simulink model "Reafference"  (R2015b)
settings: Solver=ode4  StartTime=0.0  StopTime=35.995  FixedStep=0.005  RelTol=1e-3
values from neighbouring files (symbols this model uses):
  delay = 0.25    [modelInit.m]    (also in modelInit_forward.m = 0.1)
  dt = 0.005    [modelInit.m]    (also in modelInit_forward.m)
  F = 2.0*(rand(N,dOut)-0.5)    [modelInit.m]    (also in modelInit_forward.m)
  I = 2.0*(rand(N,dIn)-0.5)    [modelInit.m]    (also in modelInit_forward.m)
  I_fore_x = infactor*(5.66+0.306*m_k-0.088*l_k)/10000    (= 0.0024252)    [modelInit.m]    (also in modelInit_forward.m)
  I_fore_y = infactor*(-64+0.95*m_k+0.34*l_k)/10000    (= 0.012004)    [modelInit.m]    (also in modelInit_forward.m)
  I_fore_z = infactor*(-67.9+0.855*m_k+0.376*l_k)/10000    (= 0.0112156)    [modelInit.m]    (also in modelInit_forward.m)
  I_hand_x = infactor*(-6.26+0.0762*m_k+0.0347*l_k)/10000    (= 0.00100322)    [modelInit.m]    (also in modelInit_forward.m)
  I_hand_y = infactor*(-19.5+0.17*m_k+0.116*l_k)/10000    (= 0.0024796)    [modelInit.m]    (also in modelInit_forward.m)
  I_hand_z = infactor*(-13.68+0.088*m_k+0.092*l_k)/10000    (= 0.0015832)    [modelInit.m]    (also in modelInit_forward.m)
  I_upper_x = (-16.9+0.662*m_k+0.0453*l_k)/10000    (= 0.00718718)    [modelInit.m]    (also in modelInit_forward.m)
  I_upper_y = (-250.7+1.56*m_k+1.512*l_k)/10000    (= 0.0247972)    [modelInit.m]    (also in modelInit_forward.m)
  I_upper_z = (-232+1.525*m_k+1.343*l_k)/10000    (= 0.0227658)    [modelInit.m]    (also in modelInit_forward.m)
  l_fore = 0.30    (= 0.3)    [modelInit.m]    (also in modelInit_forward.m)
  l_hand = 0.20    (= 0.2)    [modelInit.m]    (also in modelInit_forward.m)
  l_upper = 0.36    [modelInit.m]    (also in modelInit_forward.m)
  learn = 1    [modelLearn.m]    (also in modelLearn_forward.m; modelMorph.m = 0; modelMorph_forward.m = 0; modelVal.m = 0)
  M = full(sprandn(N,N,p)*g*1.0/sqrt(p*N))    [modelInit.m]    (also in modelInit_forward.m)
  m_fore = m_fore*wfactor    (= 1.81766)    [modelInit.m]    (also in modelInit_forward.m)
  m_hand = m_hand*wfactor    (= 0.676)    [modelInit.m]    (also in modelInit_forward.m)
  m_upper = m_upper*wfactor    (= 3.3082)    [modelInit.m]    (also in modelInit_forward.m)
  N = 1000    [modelInit.m]    (also in modelInit_forward.m)
  P0 = (1.0/alpha)*eye(N,N)    [modelInit.m]    (also in modelInit_forward.m; modelMorph.m = simOutLearn.get('P'); modelMorph_forward.m = simOutLearn.get('P'); modelVal.m = simOutLearn.get('P'))
  q0 = 0.5*randn(N,1)    [modelInit.m]    (also in modelInit_forward.m; modelMorph.m = simOutLearn.get('q'); modelMorph_forward.m = simOutLearn.get('q'); modelVal.m = simOutLearn.get('q'))
  tau = 0.01    [modelInit.m]    (also in modelInit_forward.m)
  W0 = zeros(dOut,N)    [modelInit.m]    (also in modelInit_forward.m; modelMorph.m = simOutLearn.get('W'); modelMorph_forward.m = simOutLearn.get('W'); modelVal.m = simOutLearn.get('W'))
undefined symbols (not defined in the file or in its folder): DiscIntNeverNeededParam, Muscle, MuscleLib, Newton, Raphson
undefined symbols (not defined in the file): bifactor, brfactor, trifactor
libraries: mblibv1 x26, simulink x3
settings Model: ExtModeTrigDuration=100  Creator=kbostroem  LastModifiedBy=kbostroem
settings DataIOCC: LimitDataPoints=off  SaveFinalState=on  SaveFormat=StructureWithTime  SignalLoggingSaveFormat=ModelDataLogs  SaveOutput=off  SaveState=on  StateSaveName=tmp_raccel_xout  SignalLoggingName=tmp_raccel_logsout  OutputTimes=linspace(0,20,1000)
settings OptimizationCC: ExpressionDepthLimit=2147483647  EfficientMapNaN2IntZero=off
settings DebuggingCC: UnderspecifiedInitializationDetection=Classic  MergeDetectMultiDrivingBlocksExec=none  SolverPrmCheckMsg=warning  FcnCallInpInsideContextMsg=EnableAllAsWarning  StateNameClashWarn=warning
settings HardwareCC: ProdBitPerPointer=32  ProdLargestAtomicFloat=None  ProdIntDivRoundTo=Undefined  ProdEndianess=Unspecified  ProdWordSize=32  ProdHWDeviceType=32-bit Generic  TargetBitPerLong=64  TargetBitPerPointer=64  TargetLongLongMode=on  TargetIntDivRoundTo=Zero  TargetEndianess=LittleEndian  TargetWordSize=64  TargetHWDeviceType=MATLAB Host  ProdEqTarget=off
settings RTWCC: SystemTargetFile=raccel.tlc  TemplateMakefile=raccel_default_tmf  RTWVerbose=off  RTWUseSimCustomCode=on
settings CodeAppCC: GenerateComments=off  MaxIdLength=128  MangleLength=10  SimulinkBlockComments=off
settings RaccelTargetCC: ERTMultiwordTypeDef=System defined  ERTMultiwordLength=256  GeneratePreprocessorConditionals=Disable all  ERTFirstTimeCompliant=off  MultiInstanceERTCode=off  ENABLE_SLEXEC_SSBRIDGE=0  RTWCAPIParams=off
settings ConfigComp: CovModelRefEnable=Off  CovSFcnEnable=off
settings SimscapeCC: SimscapeLogType=all  SimscapeLogDataHistory=10000
settings SimMechanicsCC: VisOnUpdateDiagram=on  LastVizWinPosition=[133 241 630 553]  CamPosition=[0.122075;1.72207;11.4539;]  CamTarget=[0.122075;1.72207;0;]  CamUpVector=[0;1;0;]  CamHeight=0.668977  VisBackgroundColor=[0.9;0.9;0.95;]  DefaultBodyColor=[1;0;0;]

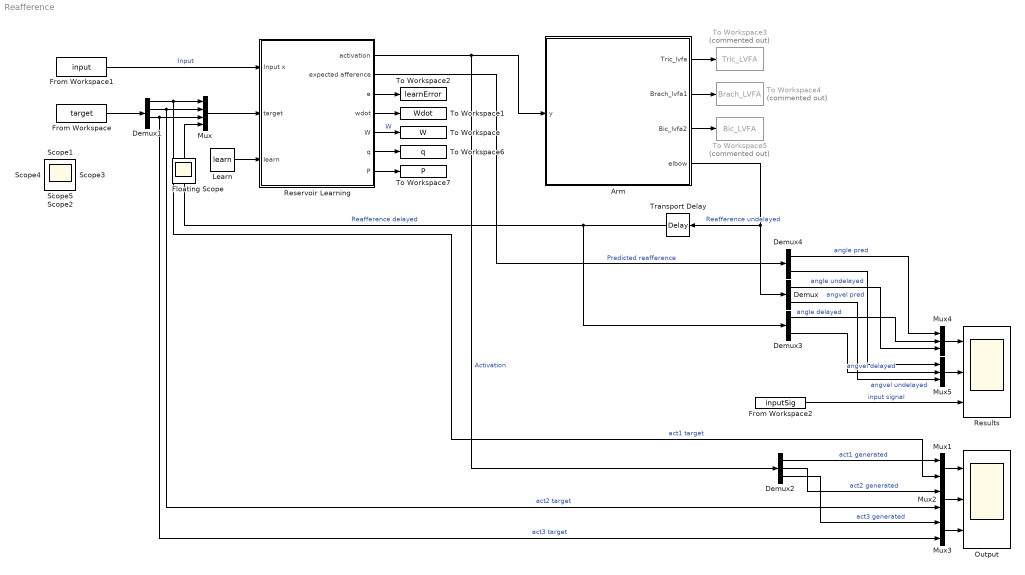
== system Reafference ==
  Arm : Subsystem
      mask Display:
      | image(imread('icons/ArmModell.jpg'));
      | 
      | port_label('output', 1, 'Tric_LVFA');
      | port_label('output', 2, 'Brach_LVFA');
      | port_label('output', 3, 'Bic_LVFA');
      | color('blue')
      | port_label('output', 4, 'Elbow Afference');
      | port_label('input', 1, 'Activation');
  Demux : Demux  Outputs=2
  Demux1 : Demux
  Demux2 : Demux  Outputs=3
  Demux3 : Demux  Outputs=2
  Demux4 : Demux  Outputs=2
  From Workspace : FromWorkspace  VariableName=target  SampleTime=dt  Interpolate=off  OutputAfterFinalValue=Cyclic repetition
  From Workspace1 : FromWorkspace  VariableName=input  SampleTime=dt  Interpolate=off  OutputAfterFinalValue=Cyclic repetition
  From Workspace2 : FromWorkspace  VariableName=inputSig  SampleTime=dt  Interpolate=off  OutputAfterFinalValue=Cyclic repetition
  Learn : Constant  Value=learn
  Mux : Mux
  Mux1 : Mux  Inputs=2
  Mux2 : Mux  Inputs=2
  Mux3 : Mux  Inputs=2
  Mux4 : Mux  Inputs=3
  Mux5 : Mux  Inputs=3
  Output : Scope  NumInputPorts=3
  Reservoir Learning : Subsystem
      mask Display:
      | image(imread('icons/liquidMotion.jpg'));
      | port_label('input', 1, 'Input x');
      | port_label('input', 2, 'Target h');
      | port_label('output', 1, 'Output y');
      | 
      | color('white')
      | port_label('input', 3, 'learn');
      | port_label('output', 2, 'Predicted reafference');
      | port_label('output', 3, 'error');
      | port_label('output', 4, 'w_dot');
      | port_label('output', 5, 'W');
      | port_label('output', 6, 'q');
      | port_label('output', 7, 'P');
  Results : Scope  NumInputPorts=3
  To Workspace : ToWorkspace  VariableName=W  SampleTime=-1
      settings: MaxDataPoints=1
  To Workspace1 : ToWorkspace  VariableName=Wdot  SampleTime=-1
      settings: MaxDataPoints=Inf
  To Workspace2 : ToWorkspace  VariableName=learnError  SampleTime=-1
      settings: MaxDataPoints=1
  To Workspace3 : ToWorkspace  Commented=on  VariableName=Tric_LVFA  SampleTime=-1
      settings: MaxDataPoints=Inf
  To Workspace4 : ToWorkspace  Commented=on  VariableName=Brach_LVFA  SampleTime=-1
      settings: MaxDataPoints=Inf
  To Workspace5 : ToWorkspace  Commented=on  VariableName=Bic_LVFA  SampleTime=-1
      settings: MaxDataPoints=Inf
  To Workspace6 : ToWorkspace  VariableName=q  SampleTime=-1
      settings: MaxDataPoints=1
  To Workspace7 : ToWorkspace  VariableName=P  SampleTime=-1
      settings: MaxDataPoints=1
  Transport Delay : TransportDelay  DelayTime=delay  InitialOutput=[130/180*pi; 0]
  Floating Scope : Scope
  Scope{,1..5} (6 alike) : Scope
  wires:
  Demux1/1 -> Mux1/2, Mux/1  "act1 target"
  Demux1/2 -> Mux2/2, Mux/2  "act2 target"
  Demux1/3 -> Mux3/2, Mux/3  "act3 target"
  Arm/4(elbow) -> Transport Delay/1, Demux/1  "Reafference undelayed"
  Mux/1 -> Reservoir Learning/2(target)
  Reservoir Learning/1(activation) -> Arm/1(y), Demux2/1  "Activation"
  Learn/1 -> Reservoir Learning/3(learn)
  From Workspace1/1 -> Reservoir Learning/1(Input x)  "Input"
  Reservoir Learning/2(expected afference) -> Demux4/1  "Predicted reafference"
  From Workspace/1 -> Demux1/1
  Reservoir Learning/5(W) -> To Workspace/1  "W"
  From Workspace2/1 -> Results/3  "input signal"
  Reservoir Learning/4(wdot) -> To Workspace1/1
  Reservoir Learning/3(e) -> To Workspace2/1
  Arm/1(Tric_lvfa) -> To Workspace3/1
  Arm/2(Brach_lvfa1) -> To Workspace4/1
  Arm/3(Bic_lvfa2) -> To Workspace5/1
  Mux1/1 -> Output/1
  Demux2/1 -> Mux1/1  "act1 generated"
  Mux2/1 -> Output/2
  Demux2/2 -> Mux2/1  "act2 generated"
  Mux3/1 -> Output/3
  Demux2/3 -> Mux3/1  "act3 generated"
  Reservoir Learning/6(q) -> To Workspace6/1
  Reservoir Learning/7(P) -> To Workspace7/1
  Transport Delay/1 -> Demux3/1, Mux/4  "Reafference delayed"
  Mux4/1 -> Results/1
  Demux/1 -> Mux4/3  "angle undelayed"
  Demux3/1 -> Mux4/2  "angle delayed"
  Demux4/1 -> Mux4/1  "angle pred"
  Mux5/1 -> Results/2
  Demux/2 -> Mux5/3  "angvel undelayed"
  Demux3/2 -> Mux5/2  "angvel delayed"
  Demux4/2 -> Mux5/1  "angvel pred"

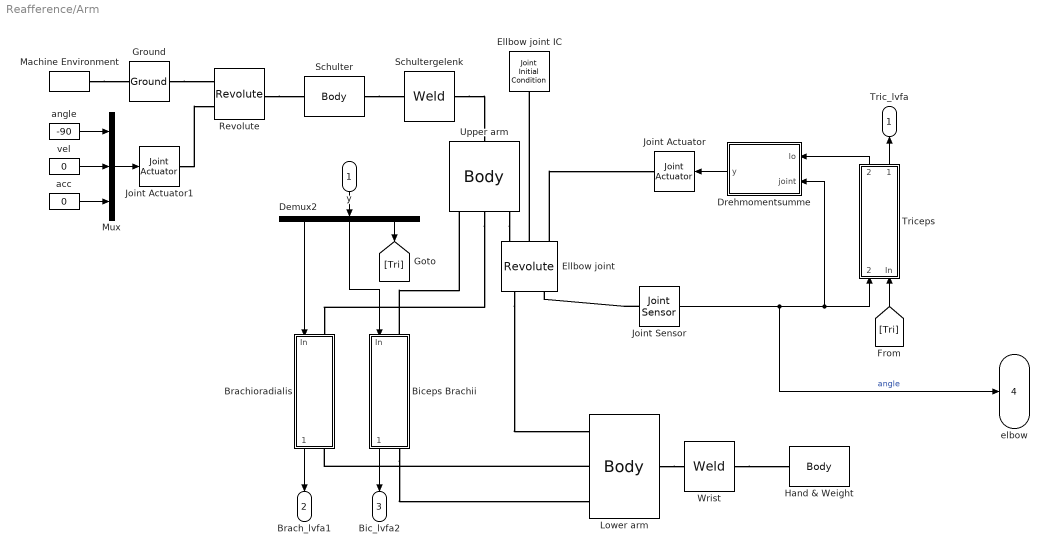
== system Reafference/Arm ==
  y : Inport
  Biceps Brachii : Subsystem  AncestorBlock=MuscleLib/Muscle  mask{PCSA=20.1*bifactor, l_0=0.185, l_tend=sqrt(l_upper^2+(0.186*l_fore)^2)-0.185, k1=0.96, k2=0.35, k3=2}
      mask prompts: l_0 "Zero-force length"; l_tend "Tendon length"
      mask init:
      | f_ecc = 1.5;
      | p_fast = 0.8;
      | l_opt = 1.2*l_0;
      | l_max = 4*l_0;
      | f_max = 25*PCSA;
      | lambda_max = 0.5*l_0;
      mask Display:
      | image(imread('icons/muscle.png'));
      | %port_label('lconn', 1, 'C1');
      | %port_label('rconn', 1, 'C2');
      | %port_label('input', 1, 'Force');
  Brachioradialis : Subsystem  AncestorBlock=MuscleLib/Muscle  mask{PCSA=9.9*brfactor, l_0=0.17, l_tend=sqrt((0.104*l_upper)^2+l_fore^2)-0.17, k1=0.96, k2=0.35, k3=2}
      mask prompts: l_0 "Zero-force length"; l_tend "Tendon length"
      mask init:
      | f_ecc = 1.5;
      | p_fast = 0.6;
      | l_opt = 1.2*l_0;
      | l_max = 4*l_0;
      | f_max = 25*PCSA;
      | lambda_max = 0.5*l_0;
      mask Display:
      | image(imread('icons/muscle.png'));
      | %port_label('lconn', 1, 'C1');
      | %port_label('rconn', 1, 'C2');
      | %port_label('input', 1, 'Force');
  Demux2 : Demux  Outputs=3
  Drehmomentsumme : MATLAB Function  TreatAsAtomicUnit=on
  Ellbow joint IC : mblibv1/Sensors &  Actuators/Joint Initial Condition  UpdateFromCAD=off  LeftPortType=blob  RightPortType=blob  PhysicalDomain=mechanical  DialogClass=InitialConditionBlock  InitialConditions=P1$false$0$m$deg$0$m/s$deg/s#P2$false$0$m$deg$0$m/s$deg/s#P3$false$0$m$deg$0$m/s$deg/s#R1$true$180-50$m$deg$0$m/s$deg/s#R2$false$0$m$deg$0$m/s$deg/s#R3$false$0$m$deg$0$m/s$deg/s#S$false$0$m$deg$0$m/s$deg/s  P1PIC=0  P1VIC=0  P2PIC=0  P2VIC=0  P3PIC=0  P3VIC=0  R1PIC=180-50  R1VIC=0  R2PIC=0  R2VIC=0  R3PIC=0  R3VIC=0  SPIC=0  SVIC=0
  Ellbow joint : mblibv1/Joints/Revolute  LConnTagsString=__newl0|SA1|SA2  RConnTagsString=__newr0|SA1  UpdateFromCAD=off  NumSAPorts=3  CutJoint=off  MarkAsCut=off  Primitives=prismatic  PrimitiveProps=R1$World$[0 0 1]$revolute  DialogClass=JointBlock  R1Axis=[0 0 1]
  Ground : mblibv1/Bodies/Ground  UpdateFromCAD=off  LeftPortType=env  RightPortType=workingframe  PhysicalDomain=Mechanical  DialogClass=GroundBlock  CoordPosition=[0 2 0]  CoordPositionUnits=m  StateVectorMgrId=-1  MachineId=[0 0]  ShowEnvPort=on  ParameterChecksum=[4130251833, 2817423392, 493878805, 1374374683]  TopologyChecksum=[1174022194, 2907012172, 545569140, 277289603]
  Hand & Weight : mblibv1/Bodies/Body  LConnTagsString=CS1  RConnTagsString=CS2  UpdateFromCAD=off  DialogClass=MechanicalBodyBlock  Mass=m_hand + 1  MassUnits=kg  InertiaUnits=kg*m^2  Inertia=[I_hand_x 0 0; 0 I_hand_y 0; 0 0 I_hand_z]  Shape=Cylinder  ShapeDims=[1 1]  ShapeUnits=m  ShapeUse=false  Density=1  DensityUnits=kg/m^3  DensityUse=false  GraphicsMode=MACHINE_DEFAULT  BodyColorSelMode=COLORPALETTE  BodyColor=[0.043137 0.51765 0.78039]  AttachedToCS=CG  CG=Left$CG$[0.369*l_hand 0 0]$CS1$CS1$m$[0 0 0]$Euler X-Y-Z$deg$WORLD$false$none  WorkingFrames=Left$CS1$[0 0 0]$Adjoining$Adjoining$m$[0 0 0]$Euler X-Y-Z$deg$WORLD$true$none#Right$CS2$[0 0 0]$CS1$CS1$m$[0 0 0]$Euler X-Y-Z$deg$WORLD$true$none  CGPos=[0.369*l_hand 0 0]  CGRot=[0 0 0]  CS0Pos=[]  CS0Rot=[]  CS1Pos=[0 0 0]  CS1Rot=[0 0 0]  CS2Pos=[0 0 0]  CS2Rot=[0 0 0]  CS3Pos=[]  CS3Rot=[]  CS4Pos=[]  CS4Rot=[]  CS5Pos=[]  CS5Rot=[]  CS6Pos=[]  CS6Rot=[]  CS7Pos=[]  CS7Rot=[]  CS8Pos=[]  CS8Rot=[]  CS9Pos=[]  CS9Rot=[]  CS10Pos=[]  CS10Rot=[]  CS11Pos=[]  CS11Rot=[]  CS12Pos=[]  CS12Rot=[]  CS13Pos=[]  CS13Rot=[]  CS14Pos=[]  CS14Rot=[]  CS15Pos=[]  CS15Rot=[]  CS16Pos=[]  CS16Rot=[]  CS17Pos=[]  CS17Rot=[]  CS18Pos=[]  CS18Rot=[]  CS19Pos=[]  CS19Rot=[]  CS20Pos=[]  CS20Rot=[]
  Joint Actuator : mblibv1/Sensors &  Actuators/Joint Actuator  UpdateFromCAD=off  PhysicalDomain=Mechanical  PortType=blob  ActuationStyle=Force  AngleUnits=deg  ArcVelocityUnits=deg/s  ArcAccelerationUnits=deg/s^2  CoordPositionUnits=m  VelocityUnits=m/s  AccelerationUnits=m/s^2  ForceUnits=N  TorqueUnits=N*m  ActiveIO=on  Width=1  DialogClass=MechanicalActuatorBlock  Primitive=R1  ReferenceFrame=Absolute (World)
  Joint Actuator1 : mblibv1/Sensors &  Actuators/Joint Actuator  UpdateFromCAD=off  PhysicalDomain=Mechanical  PortType=blob  ActuationStyle=Motion  AngleUnits=deg  ArcVelocityUnits=deg/s  ArcAccelerationUnits=deg/s^2  CoordPositionUnits=m  VelocityUnits=m/s  AccelerationUnits=m/s^2  ForceUnits=N  TorqueUnits=N*m  ActiveIO=on  Width=3  DialogClass=MechanicalActuatorBlock  Primitive=R1  ReferenceFrame=Absolute (World)
  Joint Sensor : mblibv1/Sensors &  Actuators/Joint Sensor  UpdateFromCAD=off  PhysicalDomain=Mechanical  PortType=blob  Muxed=on  Pose=off  Angle=on  AngleUnits=rad  ArcVelocity=on  ArcVelocityUnits=rad/s  ArcAcceleration=off  ArcAccelerationUnits=deg/s^2  CoordPosition=on  CoordPositionUnits=m  Velocity=off  VelocityUnits=m/s  Acceleration=off  AccelerationUnits=m/s^2  Quaternion=on  QuaternionDT=off  QuaternionDDT=off  QuaternionUnits=off  OutputVector=[1]  ActiveIO=on  Width=2  DialogClass=MechanicalSensorBlock  Primitive=R1  Force=off  ForceUnits=N  Torque=off  TorqueUnits=N*m  ReferenceFrame=Absolute (World)  ReactionSensedSide=Base  ReactionReferenceFrame=Absolute (World)  ReactionForce=off  ReactionForceUnits=N  ReactionMoment=off  ReactionMomentUnits=N*m
  Lower arm : mblibv1/Bodies/Body  LConnTagsString=CS1|CS6|CS3  RConnTagsString=CS2  UpdateFromCAD=off  DialogClass=MechanicalBodyBlock  Mass=m_fore  MassUnits=kg  InertiaUnits=kg*m^2  Inertia=[I_fore_x 0 0; 0 I_fore_y 0; 0 0 I_fore_z]  Shape=Cylinder  ShapeDims=[1 1]  ShapeUnits=m  ShapeUse=false  Density=1  DensityUnits=kg/m^3  DensityUse=false  GraphicsMode=MACHINE_DEFAULT  BodyColorSelMode=COLORPALETTE  BodyColor=[1 0 0]  AttachedToCS=CG  CG=Left$CG$[0.4274*l_fore 0 0]$CS1$CS1$m$[0 0 0]$Euler X-Y-Z$deg$WORLD$false$none  WorkingFrames=Left$CS1$[0 0 0]$Adjoining$Adjoining$m$[0 0 0]$Euler X-Y-Z$deg$WORLD$true$none#Left$CS6$[l_fore 0 0]$CS1$CS1$m$[0 0 0]$Euler X-Y-Z$deg$WORLD$true$none#Right$CS2$[l_fore 0 0]$CS1$CS1$m$[0 0 0]$Euler X-Y-Z$deg$WORLD$true$none#Left$CS3$[0.186*l_fore 0 0]$CS1$CS1$m$[0 0 0]$Euler X-Y-Z$deg$WORLD$true$none#Left$CS4$[-0.05*l_fore 0 0]$CS1$CS1$m$[0 0 0]$Euler X-Y-Z$deg$WORLD$false$none#Left$CS5$[-0.05*l_fore 0 0]$CS1$CS1$m$[0 0 0]$Euler X-Y-Z$deg$WORLD$false$none  CGPos=[0.4274*l_fore 0 0]  CGRot=[0 0 0]  CS0Pos=[]  CS0Rot=[]  CS1Pos=[0 0 0]  CS1Rot=[0 0 0]  CS2Pos=[l_fore 0 0]  CS2Rot=[0 0 0]  CS3Pos=[0.186*l_fore 0 0]  CS3Rot=[0 0 0]  CS4Pos=[-0.05*l_fore 0 0]  CS4Rot=[0 0 0]  CS5Pos=[-0.05*l_fore 0 0]  CS5Rot=[0 0 0]  CS6Pos=[l_fore 0 0]  CS6Rot=[0 0 0]  CS7Pos=[]  CS7Rot=[]  CS8Pos=[]  CS8Rot=[]  CS9Pos=[]  CS9Rot=[]  CS10Pos=[]  CS10Rot=[]  CS11Pos=[]  CS11Rot=[]  CS12Pos=[]  CS12Rot=[]  CS13Pos=[]  CS13Rot=[]  CS14Pos=[]  CS14Rot=[]  CS15Pos=[]  CS15Rot=[]  CS16Pos=[]  CS16Rot=[]  CS17Pos=[]  CS17Rot=[]  CS18Pos=[]  CS18Rot=[]  CS19Pos=[]  CS19Rot=[]  CS20Pos=[]  CS20Rot=[]
  Machine Environment : mblibv1/Bodies/Machine Environment  PortType=env  PhysicalDomain=Mechanical  DialogTemplateClass=MECH.MachineEnvironment  SyncWhenCopied=off  Gravity=[0 -9.81 0]  GravityUnits=m/s^2  GravityAsSignal=off  Dimensionality=Auto-detect  AnalysisType=Forward dynamics  LinearAssemblyTolerance=1e-3  LinearAssemblyToleranceUnits=m  AngularAssemblyTolerance=1e-3  AngularAssemblyToleranceUnits=rad  ConstraintSolverType=Stabilizing  ConstraintRelTolerance=1e-4  ConstraintAbsTolerance=1e-4  UseRobustSingularityHandling=off  RedundancyAnalysisToleranceType=Automatically select tolerance  RedundancyAnalysisTolerance=1e-14  StatePerturbationType=Fixed  PerturbationSize=1e-5  VisualizeMachine=on  BodyVisualizationType=Equivalent ellipsoid from mass properties  BodyColorSelMode=Specify  DefaultBodyColor=[1 0 0]
  Mux : Mux  Inputs=3
  Revolute : mblibv1/Joints/Revolute  LConnTagsString=__newl0|SA1  RConnTagsString=__newr0  UpdateFromCAD=off  NumSAPorts=1  CutJoint=off  MarkAsCut=off  Primitives=prismatic  PrimitiveProps=R1$World$[0 0 1]$revolute  DialogClass=JointBlock  R1Axis=[0 0 1]
  Schulter : mblibv1/Bodies/Body  LConnTagsString=CS1  RConnTagsString=CS2  UpdateFromCAD=off  DialogClass=MechanicalBodyBlock  Mass=1  MassUnits=kg  InertiaUnits=kg*m^2  Inertia=eye(3)*0.001  Shape=Cylinder  ShapeDims=[1 1]  ShapeUnits=m  ShapeUse=false  Density=1  DensityUnits=kg/m^3  DensityUse=false  GraphicsMode=EQELLIPSE  BodyColorSelMode=COLORPALETTE  BodyColor=[0.043137 0.51765 0.78039]  AttachedToCS=CG  CG=Left$CG$[0 0 0]$CS1$CS1$m$[0 0 0]$Euler X-Y-Z$deg$WORLD$false$none  WorkingFrames=Left$CS1$[0 0 0]$Adjoining$Adjoining$m$[0 0 0]$Euler X-Y-Z$deg$WORLD$true$none#Right$CS2$[0 0 0]$CS1$CS1$m$[0 0 0]$Euler X-Y-Z$deg$WORLD$true$none#Left$CS6$[0 0 -0.05]$CS1$CS1$m$[0 0 0]$Euler X-Y-Z$deg$WORLD$false$none  CGPos=[0 0 0]  CGRot=[0 0 0]  CS0Pos=[]  CS0Rot=[]  CS1Pos=[0 0 0]  CS1Rot=[0 0 0]  CS2Pos=[0 0 0]  CS2Rot=[0 0 0]  CS3Pos=[]  CS3Rot=[]  CS4Pos=[]  CS4Rot=[]  CS5Pos=[]  CS5Rot=[]  CS6Pos=[0 0 -0.05]  CS6Rot=[0 0 0]  CS7Pos=[]  CS7Rot=[]  CS8Pos=[]  CS8Rot=[]  CS9Pos=[]  CS9Rot=[]  CS10Pos=[]  CS10Rot=[]  CS11Pos=[]  CS11Rot=[]  CS12Pos=[]  CS12Rot=[]  CS13Pos=[]  CS13Rot=[]  CS14Pos=[]  CS14Rot=[]  CS15Pos=[]  CS15Rot=[]  CS16Pos=[]  CS16Rot=[]  CS17Pos=[]  CS17Rot=[]  CS18Pos=[]  CS18Rot=[]  CS19Pos=[]  CS19Rot=[]  CS20Pos=[]  CS20Rot=[]
  Schultergelenk : mblibv1/Joints/Weld  LConnTagsString=__newl0  RConnTagsString=__newr0  UpdateFromCAD=off  NumSAPorts=0  CutJoint=off  MarkAsCut=off  Primitives=weld  PrimitiveProps=W$World$[0 0 0]$weld  DialogClass=JointBlock  WAxis=[0 0 0]
  Triceps : Subsystem  AncestorBlock=MuscleLib/Muscle  mask{PCSA=28.9*trifactor, l_0=0.21, l_tend=sqrt((0.2*l_fore)^2+l_upper^2)-0.21, k1=0.96, k2=0.35, k3=2, l_fore=l_fore}
      mask prompts: l_0 "Zero-force length"; l_tend "Tendon length"
      mask init:
      | f_ecc = 1.5;
      | p_fast = 0.8;
      | l_opt = 1.2*l_0;
      | l_max = 4*l_0;
      | f_max = 25*PCSA;
      | lambda_max = 0.5*l_0;
      mask Display:
      | image(imread('icons/muscle.png'));
      | %port_label('lconn', 1, 'C1');
      | %port_label('rconn', 1, 'C2');
      | %port_label('input', 1, 'Force');
  Upper arm : mblibv1/Bodies/Body  LConnTagsString=CS1  RConnTagsString=CS3|CS5|CS2  UpdateFromCAD=off  DialogClass=MechanicalBodyBlock  Mass=m_upper  MassUnits=kg  InertiaUnits=kg*m^2  Inertia=[I_upper_x 0 0; 0 I_upper_y 0; 0 0 I_upper_z]  Shape=Cylinder  ShapeDims=[1 1]  ShapeUnits=m  ShapeUse=false  Density=1  DensityUnits=kg/m^3  DensityUse=false  GraphicsMode=MACHINE_DEFAULT  BodyColorSelMode=COLORPALETTE  BodyColor=[1 0 0]  AttachedToCS=CG  CG=Left$CG$[0.4498*l_upper 0 0]$CS1$CS1$m$[0 0 0]$Euler X-Y-Z$deg$WORLD$false$none  WorkingFrames=Left$CS1$[0 0 0]$Adjoining$Adjoining$m$[0 0 0]$Euler X-Y-Z$deg$WORLD$true$none#Right$CS4$[0.196*l_upper 0 0]$CS1$CS1$m$[0 0 0]$Euler X-Y-Z$deg$WORLD$false$none#Right$CS3$[0 0 0]$CS1$CS1$m$[0 0 0]$Euler X-Y-Z$deg$WORLD$true$none#Right$CS5$[0.896*l_upper 0 0]$CS1$CS1$m$[0 0 0]$Euler X-Y-Z$deg$WORLD$true$none#Right$CS2$[l_upper 0 0]$CS1$CS1$m$[0 0 0]$Euler X-Y-Z$deg$WORLD$true$none  CGPos=[0.4498*l_upper 0 0]  CGRot=[0 0 0]  CS0Pos=[]  CS0Rot=[]  CS1Pos=[0 0 0]  CS1Rot=[0 0 0]  CS2Pos=[l_upper 0 0]  CS2Rot=[0 0 0]  CS3Pos=[0 0 0]  CS3Rot=[0 0 0]  CS4Pos=[0.196*l_upper 0 0]  CS4Rot=[0 0 0]  CS5Pos=[0.896*l_upper 0 0]  CS5Rot=[0 0 0]  CS6Pos=[]  CS6Rot=[]  CS7Pos=[]  CS7Rot=[]  CS8Pos=[]  CS8Rot=[]  CS9Pos=[]  CS9Rot=[]  CS10Pos=[]  CS10Rot=[]  CS11Pos=[]  CS11Rot=[]  CS12Pos=[]  CS12Rot=[]  CS13Pos=[]  CS13Rot=[]  CS14Pos=[]  CS14Rot=[]  CS15Pos=[]  CS15Rot=[]  CS16Pos=[]  CS16Rot=[]  CS17Pos=[]  CS17Rot=[]  CS18Pos=[]  CS18Rot=[]  CS19Pos=[]  CS19Rot=[]  CS20Pos=[]  CS20Rot=[]
  Wrist : mblibv1/Joints/Weld  LConnTagsString=__newl0  RConnTagsString=__newr0  UpdateFromCAD=off  NumSAPorts=0  CutJoint=off  MarkAsCut=off  Primitives=weld  PrimitiveProps=W$World$[0 0 0]$weld  DialogClass=JointBlock  WAxis=[0 0 0]
  acc : Constant  Value=0
  angle : Constant  Value=-90
  vel : Constant  Value=0
  Tric_lvfa : Outport
  Brach_lvfa1 : Outport  Port=2
  Bic_lvfa2 : Outport  Port=3
  elbow : Outport  Port=4
  wires:
  Joint Sensor/1 -> Drehmomentsumme/2(joint), Triceps/2(elbow angle), elbow/1  "angle"
  angle/1 -> Mux/1
  vel/1 -> Mux/2
  acc/1 -> Mux/3
  Mux/1 -> Joint Actuator1/1
  Drehmomentsumme/1(y) -> Joint Actuator/1
  Triceps/2("Drehmoment ") -> Drehmomentsumme/1(lo)
  Demux2/1 -> Brachioradialis/1(In)
  Demux2/2 -> Biceps Brachii/1(In)
  y/1 -> Demux2/1
  Triceps/1(sensorOut) -> Tric_lvfa/1
  Brachioradialis/1(sensorOut) -> Brach_lvfa1/1
  Biceps Brachii/1(sensorOut) -> Bic_lvfa2/1
  Demux2/3 -> [Tri]
  [Tri] -> Triceps/1(In)
  connections:
  Biceps Brachii/LConn1 -- Upper arm/RConn1
  Biceps Brachii/RConn1 -- Lower arm/LConn3
  Upper arm/RConn2 -- Brachioradialis/LConn1
  Lower arm/LConn2 -- Brachioradialis/RConn1
  Ellbow joint/LConn2 -- Ellbow joint IC/RConn1
  Upper arm/RConn3 -- Ellbow joint/LConn1
  Ellbow joint/LConn3 -- Joint Actuator/RConn1
  Ellbow joint/RConn1 -- Lower arm/LConn1
  Joint Sensor/LConn1 -- Ellbow joint/RConn2
  Machine Environment/RConn1 -- Ground/LConn1
  Ground/RConn1 -- Revolute/LConn1
  Wrist/RConn1 -- Hand & Weight/LConn1
  Joint Actuator1/RConn1 -- Revolute/LConn2
  Lower arm/RConn1 -- Wrist/LConn1
  Revolute/RConn1 -- Schulter/LConn1
  Schulter/RConn1 -- Schultergelenk/LConn1
  Schultergelenk/RConn1 -- Upper arm/LConn1

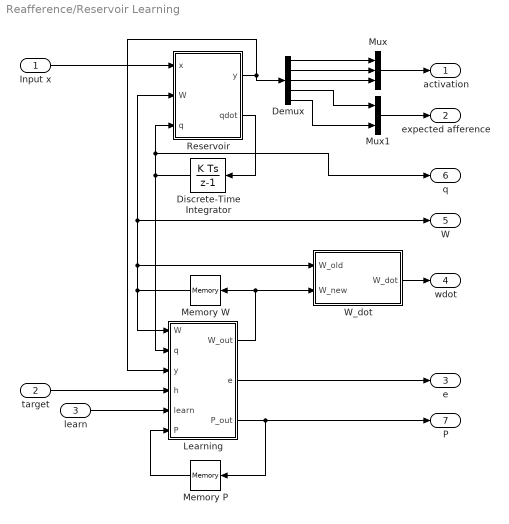
== system Reafference/Reservoir Learning ==
  Input x : Inport
  target : Inport  Port=2
  learn : Inport  Port=3
  Demux : Demux  Outputs=5
  Discrete-Time Integrator : DiscreteIntegrator  InitialCondition=q0  SampleTime=dt  ICPrevOutput=DiscIntNeverNeededParam  ICPrevScaledInput=DiscIntNeverNeededParam
  Learning : MATLAB Function  TreatAsAtomicUnit=on
  Memory P : Memory  X0=P0
  Memory W : Memory  X0=W0
  Mux : Mux  Inputs=3
  Mux1 : Mux  Inputs=2
  Reservoir : MATLAB Function  TreatAsAtomicUnit=on
  W_dot : MATLAB Function  TreatAsAtomicUnit=on
  activation : Outport
  expected afference : Outport  Port=2
  e : Outport  Port=3
  wdot : Outport  Port=4
  W : Outport  Port=5
  q : Outport  Port=6
  P : Outport  Port=7
  wires:
  Discrete-Time Integrator/1 -> Learning/2(q), q/1, Reservoir/3(q)
  Reservoir/2(qdot) -> Discrete-Time Integrator/1
  Input x/1 -> Reservoir/1(x)
  Learning/1(W_out) -> W_dot/2(W_new), Memory W/1
  Memory W/1 -> Learning/1(W), Reservoir/2(W), W/1, W_dot/1(W_old)
  Learning/3(P_out) -> Memory P/1, P/1
  Memory P/1 -> Learning/6(P)
  target/1 -> Learning/4(h)
  Learning/2(e) -> e/1
  learn/1 -> Learning/5(learn)
  Reservoir/1(y) -> Learning/3(y), Demux/1
  Demux/1 -> Mux/1
  Demux/2 -> Mux/2
  Demux/3 -> Mux/3
  Mux/1 -> activation/1
  Demux/4 -> Mux1/1
  W_dot/1(W_dot) -> wdot/1
  Demux/5 -> Mux1/2
  Mux1/1 -> expected afference/1

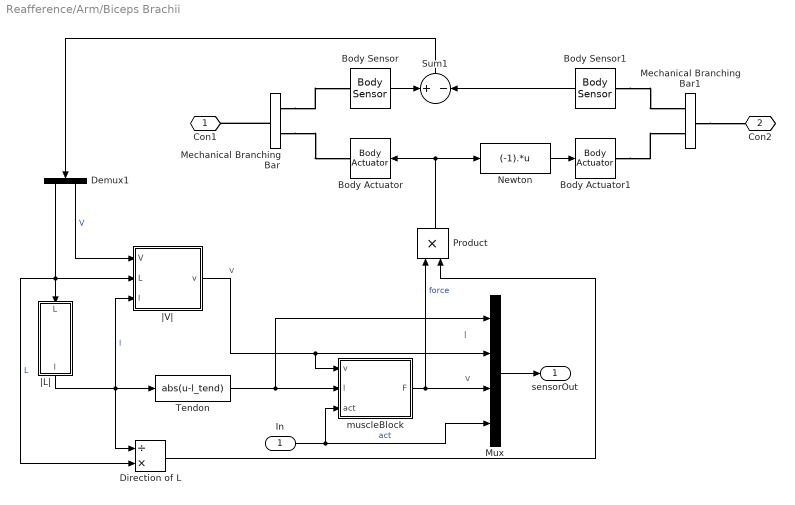
== system Reafference/Arm/Biceps Brachii ==
  note: l
  note: v
  note: v
  In : Inport
  Body Actuator : mblibv1/Sensors &  Actuators/Body Actuator  UpdateFromCAD=off  PhysicalDomain=Mechanical  PortType=blob  ActuationStyle=Force  AngleUnits=deg  ArcVelocityUnits=deg/s  ArcAccelerationUnits=deg/s^2  CoordPositionUnits=m  VelocityUnits=m/s  AccelerationUnits=m/s^2  ForceUnits=N  TorqueUnits=N-m  ActiveIO=on  Width=3  DialogClass=MechanicalActuatorBlock  ReferenceFrame=Absolute (INERTIAL)  Angle=off  CoordPosition=on  Force=on  Torque=off
  Body Actuator1 : mblibv1/Sensors &  Actuators/Body Actuator  UpdateFromCAD=off  PhysicalDomain=Mechanical  PortType=blob  ActuationStyle=Force  AngleUnits=deg  ArcVelocityUnits=deg/s  ArcAccelerationUnits=deg/s^2  CoordPositionUnits=m  VelocityUnits=m/s  AccelerationUnits=m/s^2  ForceUnits=N  TorqueUnits=N*m  ActiveIO=on  Width=3  DialogClass=MechanicalActuatorBlock  ReferenceFrame=Absolute (World)  Angle=off  CoordPosition=on  Force=on  Torque=off
  Body Sensor : mblibv1/Sensors &  Actuators/Body Sensor  UpdateFromCAD=off  PhysicalDomain=Mechanical  PortType=blob  Muxed=on  Pose=off  Angle=on  AngleUnits=deg  ArcVelocity=off  ArcVelocityUnits=deg/s  ArcAcceleration=off  ArcAccelerationUnits=deg/s^2  CoordPosition=on  CoordPositionUnits=m  Velocity=on  VelocityUnits=m/s  Acceleration=off  AccelerationUnits=m/s^2  Quaternion=on  QuaternionDT=off  QuaternionDDT=off  QuaternionUnits=deg  OutputVector=[ 3 3 ]  ActiveIO=on  Width=6  DialogClass=MechanicalSensorBlock  ReferenceFrame=Absolute (World)
  Body Sensor1 : mblibv1/Sensors &  Actuators/Body Sensor  UpdateFromCAD=off  PhysicalDomain=Mechanical  PortType=blob  Muxed=on  Pose=off  Angle=on  AngleUnits=deg  ArcVelocity=off  ArcVelocityUnits=deg/s  ArcAcceleration=off  ArcAccelerationUnits=deg/s^2  CoordPosition=on  CoordPositionUnits=m  Velocity=on  VelocityUnits=m/s  Acceleration=off  AccelerationUnits=m/s^2  Quaternion=on  QuaternionDT=off  QuaternionDDT=off  QuaternionUnits=deg  OutputVector=[ 3 3 ]  ActiveIO=on  Width=6  DialogClass=MechanicalSensorBlock  ReferenceFrame=Absolute (World)
  Demux1 : Demux  Outputs=2
  Direction of L : Product  Inputs=/*
  Mechanical Branching Bar : mblibv1/Utilities/Mechanical Branching Bar  LConnTagsString=_newl0  RConnTagsString=__newr0|SA2  UpdateFromCAD=off  DialogClass=MechanicalBranchingBarBlock  NumSAPorts=2
  Mechanical Branching Bar1 : mblibv1/Utilities/Mechanical Branching Bar  LConnTagsString=_newl0  RConnTagsString=__newr0|SA2  UpdateFromCAD=off  DialogClass=MechanicalBranchingBarBlock  NumSAPorts=2
  Mux : Mux
  Newton : MATLABFcn  MATLABFcn=(-1).*u
  Product : Product  RndMeth=Zero
  Sum1 : Sum  Inputs=+-  SaturateOnIntegerOverflow=on
  Tendon : Fcn  Expr=abs(u-l_tend)
  muscleBlock : Subsystem  mask{PCSA=PCSA, l_0=l_0, p_fast=p_fast, f_ecc=f_ecc, l_opt=l_opt, l_max=l_max, f_max=f_max, lambda_max=lambda_max, l_tend=l_tend, k1=k1, k2=k2, k3=k3}
      mask init:
      | f_iso = 25*PCSA;
      | v_max = (6+p_fast*10)*l_opt;
      | 
      | a = 0.25*f_iso;
      | b = 0.25*v_max;
      | c = b*(f_iso+a);
      | 
      | a_ecc = f_ecc*f_iso; 
      | b_ecc = (a_ecc-f_iso)*b^2/c; 
      | c_ecc = (a_ecc-f_iso)*b_ecc;
      mask Display:
      | image(imread('icons/muscle.png'));
      | port_label('input', 3, 'Act');
      | port_label('input', 2, 'l');
      | port_label('input', 1, 'v');
      | port_label('output', 1, 'Force');
  |L| : Subsystem
  |V| : Subsystem
  Con1 : PMIOPort  Port=1  Side=Left
  Con2 : PMIOPort  Port=2  Side=Right
  sensorOut : Outport
  wires:
  muscleBlock/1(F) -> Mux/3, Product/1  "force"
  Newton/1 -> Body Actuator1/1
  Sum1/1 -> Demux1/1
  Body Sensor/1 -> Sum1/1
  Demux1/2 -> |V|/1(V)  "V"
  |V|/1(v) -> Mux/2, muscleBlock/1(v)
  Mux/1 -> sensorOut/1
  Product/1 -> Newton/1, Body Actuator/1
  Body Sensor1/1 -> Sum1/2
  Tendon/1 -> Mux/1, muscleBlock/2(l)
  In/1 -> Mux/4, muscleBlock/3(act)  "act"
  Direction of L/1 -> Product/2
  Demux1/1 -> Direction of L/2, |L|/1(L), |V|/2(L)  "L"
  |L|/1(l) -> Direction of L/1, Tendon/1, |V|/3(l)  "l"
  connections:
  Mechanical Branching Bar/LConn1 -- Con1/RConn1
  Body Sensor1/LConn1 -- Mechanical Branching Bar1/RConn1
  Mechanical Branching Bar/RConn1 -- Body Sensor/LConn1
  Mechanical Branching Bar1/LConn1 -- Con2/RConn1
  Mechanical Branching Bar/RConn2 -- Body Actuator/RConn1
  Body Actuator1/RConn1 -- Mechanical Branching Bar1/RConn2

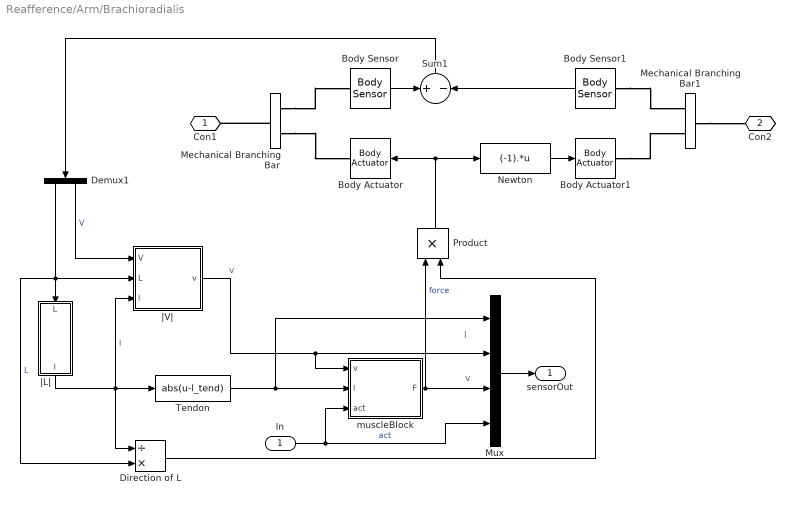
== system Reafference/Arm/Brachioradialis ==
  note: l
  note: v
  note: v
  In : Inport
  Body Actuator : mblibv1/Sensors &  Actuators/Body Actuator  UpdateFromCAD=off  PhysicalDomain=Mechanical  PortType=blob  ActuationStyle=Force  AngleUnits=deg  ArcVelocityUnits=deg/s  ArcAccelerationUnits=deg/s^2  CoordPositionUnits=m  VelocityUnits=m/s  AccelerationUnits=m/s^2  ForceUnits=N  TorqueUnits=N-m  ActiveIO=on  Width=3  DialogClass=MechanicalActuatorBlock  ReferenceFrame=Absolute (INERTIAL)  Angle=off  CoordPosition=on  Force=on  Torque=off
  Body Actuator1 : mblibv1/Sensors &  Actuators/Body Actuator  UpdateFromCAD=off  PhysicalDomain=Mechanical  PortType=blob  ActuationStyle=Force  AngleUnits=deg  ArcVelocityUnits=deg/s  ArcAccelerationUnits=deg/s^2  CoordPositionUnits=m  VelocityUnits=m/s  AccelerationUnits=m/s^2  ForceUnits=N  TorqueUnits=N*m  ActiveIO=on  Width=3  DialogClass=MechanicalActuatorBlock  ReferenceFrame=Absolute (World)  Angle=off  CoordPosition=on  Force=on  Torque=off
  Body Sensor : mblibv1/Sensors &  Actuators/Body Sensor  UpdateFromCAD=off  PhysicalDomain=Mechanical  PortType=blob  Muxed=on  Pose=off  Angle=on  AngleUnits=deg  ArcVelocity=off  ArcVelocityUnits=deg/s  ArcAcceleration=off  ArcAccelerationUnits=deg/s^2  CoordPosition=on  CoordPositionUnits=m  Velocity=on  VelocityUnits=m/s  Acceleration=off  AccelerationUnits=m/s^2  Quaternion=on  QuaternionDT=off  QuaternionDDT=off  QuaternionUnits=deg  OutputVector=[ 3 3 ]  ActiveIO=on  Width=6  DialogClass=MechanicalSensorBlock  ReferenceFrame=Absolute (World)
  Body Sensor1 : mblibv1/Sensors &  Actuators/Body Sensor  UpdateFromCAD=off  PhysicalDomain=Mechanical  PortType=blob  Muxed=on  Pose=off  Angle=on  AngleUnits=deg  ArcVelocity=off  ArcVelocityUnits=deg/s  ArcAcceleration=off  ArcAccelerationUnits=deg/s^2  CoordPosition=on  CoordPositionUnits=m  Velocity=on  VelocityUnits=m/s  Acceleration=off  AccelerationUnits=m/s^2  Quaternion=on  QuaternionDT=off  QuaternionDDT=off  QuaternionUnits=deg  OutputVector=[ 3 3 ]  ActiveIO=on  Width=6  DialogClass=MechanicalSensorBlock  ReferenceFrame=Absolute (World)
  Demux1 : Demux  Outputs=2
  Direction of L : Product  Inputs=/*
  Mechanical Branching Bar : mblibv1/Utilities/Mechanical Branching Bar  LConnTagsString=_newl0  RConnTagsString=__newr0|SA2  UpdateFromCAD=off  DialogClass=MechanicalBranchingBarBlock  NumSAPorts=2
  Mechanical Branching Bar1 : mblibv1/Utilities/Mechanical Branching Bar  LConnTagsString=_newl0  RConnTagsString=__newr0|SA2  UpdateFromCAD=off  DialogClass=MechanicalBranchingBarBlock  NumSAPorts=2
  Mux : Mux
  Newton : MATLABFcn  MATLABFcn=(-1).*u
  Product : Product  RndMeth=Zero
  Sum1 : Sum  Inputs=+-  SaturateOnIntegerOverflow=on
  Tendon : Fcn  Expr=abs(u-l_tend)
  muscleBlock : Subsystem  mask{PCSA=PCSA, l_0=l_0, p_fast=p_fast, f_ecc=f_ecc, l_opt=l_opt, l_max=l_max, f_max=f_max, lambda_max=lambda_max, l_tend=l_tend, k1=k1, k2=k2, k3=k3}
      mask init:
      | f_iso = 25*PCSA;
      | v_max = (6+p_fast*10)*l_opt;
      | 
      | a = 0.25*f_iso;
      | b = 0.25*v_max;
      | c = b*(f_iso+a);
      | 
      | a_ecc = f_ecc*f_iso; 
      | b_ecc = (a_ecc-f_iso)*b^2/c; 
      | c_ecc = (a_ecc-f_iso)*b_ecc;
      mask Display:
      | image(imread('icons/muscle.png'));
      | port_label('input', 3, 'Act');
      | port_label('input', 2, 'l');
      | port_label('input', 1, 'v');
      | port_label('output', 1, 'Force');
  |L| : Subsystem
  |V| : Subsystem
  Con1 : PMIOPort  Port=1  Side=Left
  Con2 : PMIOPort  Port=2  Side=Right
  sensorOut : Outport
  wires:
  muscleBlock/1(F) -> Mux/3, Product/1  "force"
  Newton/1 -> Body Actuator1/1
  Sum1/1 -> Demux1/1
  Body Sensor/1 -> Sum1/1
  Demux1/2 -> |V|/1(V)  "V"
  |V|/1(v) -> Mux/2, muscleBlock/1(v)
  Mux/1 -> sensorOut/1
  Product/1 -> Newton/1, Body Actuator/1
  Body Sensor1/1 -> Sum1/2
  Tendon/1 -> Mux/1, muscleBlock/2(l)
  In/1 -> Mux/4, muscleBlock/3(act)  "act"
  Direction of L/1 -> Product/2
  Demux1/1 -> Direction of L/2, |L|/1(L), |V|/2(L)  "L"
  |L|/1(l) -> Direction of L/1, Tendon/1, |V|/3(l)  "l"
  connections:
  Mechanical Branching Bar/LConn1 -- Con1/RConn1
  Body Sensor1/LConn1 -- Mechanical Branching Bar1/RConn1
  Mechanical Branching Bar/RConn1 -- Body Sensor/LConn1
  Mechanical Branching Bar1/LConn1 -- Con2/RConn1
  Mechanical Branching Bar/RConn2 -- Body Actuator/RConn1
  Body Actuator1/RConn1 -- Mechanical Branching Bar1/RConn2

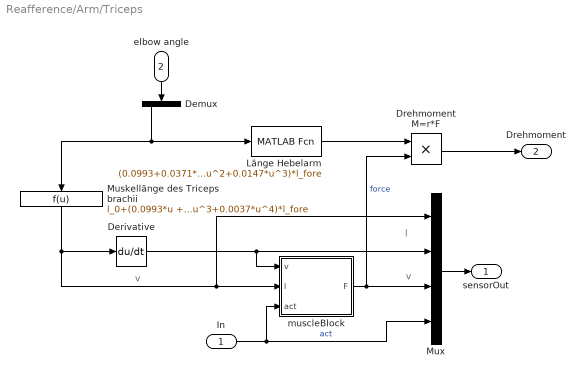
== system Reafference/Arm/Triceps ==
  note: l
  note: v
  note: v
  In : Inport
  elbow angle : Inport  Port=2
  Demux : Demux  Outputs=2
  Derivative : Derivative
  Drehmoment M=r*F : Product  RndMeth=Zero
  Länge Hebelarm : MATLABFcn  MATLABFcn=(0.0993+0.0371*u-0.0524*u^2+0.0147*u^3)*l_fore  OutputSignalType=real
  Muskellänge des Triceps brachii : Fcn  Expr=l_0+(0.0993*u +0.0186*u^2-0.0175*u^3+0.0037*u^4)*l_fore
  Mux : Mux
  muscleBlock : Subsystem  mask{PCSA=PCSA, l_0=l_0, p_fast=p_fast, f_ecc=f_ecc, l_opt=l_opt, l_max=l_max, f_max=f_max, lambda_max=lambda_max, l_tend=l_tend, k1=k1, k2=k2, k3=k3}
      mask init:
      | f_iso = 25*PCSA;
      | v_max = (6+p_fast*10)*l_opt;
      | 
      | a = 0.25*f_iso;
      | b = 0.25*v_max;
      | c = b*(f_iso+a);
      | 
      | a_ecc = f_ecc*f_iso; 
      | b_ecc = (a_ecc-f_iso)*b^2/c; 
      | c_ecc = (a_ecc-f_iso)*b_ecc;
      mask Display:
      | image(imread('icons/muscle.png'));
      | port_label('input', 3, 'Act');
      | port_label('input', 2, 'l');
      | port_label('input', 1, 'v');
      | port_label('output', 1, 'Force');
  sensorOut : Outport
  "Drehmoment " : Outport  Port=2
  wires:
  muscleBlock/1(F) -> Mux/3, Drehmoment M=r*F/2  "force"
  Derivative/1 -> Mux/2, muscleBlock/1(v)
  Mux/1 -> sensorOut/1
  Muskellänge des Triceps brachii/1 -> Mux/1, muscleBlock/2(l), Derivative/1
  In/1 -> Mux/4, muscleBlock/3(act)  "act"
  Drehmoment M=r*F/1 -> "Drehmoment "/1
  Länge Hebelarm/1 -> Drehmoment M=r*F/1
  elbow angle/1 -> Demux/1
  Demux/1 -> Länge Hebelarm/1, Muskellänge des Triceps brachii/1

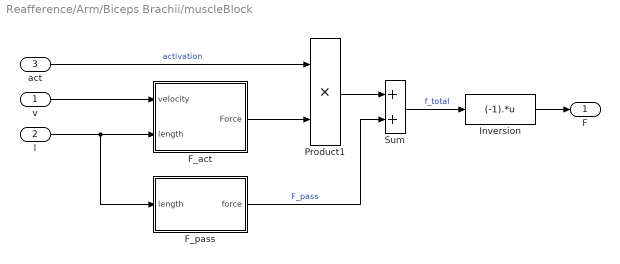
== system Reafference/Arm/Biceps Brachii/muscleBlock ==
  v : Inport
  l : Inport  Port=2
  act : Inport  Port=3
  F_act : Subsystem  Description=active part of the force
  F_pass : Subsystem
  Inversion : MATLABFcn  MATLABFcn=(-1).*u
  Product1 : Product  RndMeth=Zero
  Sum : Sum
  F : Outport
  wires:
  v/1 -> F_act/1(velocity)
  l/1 -> F_pass/1(length), F_act/2(length)
  F_pass/1(force) -> Sum/2  "F_pass"
  Inversion/1 -> F/1
  Sum/1 -> Inversion/1  "f_total"
  Product1/1 -> Sum/1
  F_act/1(Force) -> Product1/2
  act/1 -> Product1/1  "activation"

== system Reafference/Arm/Biceps Brachii/|L| ==
  L : Inport
  Dot Product1 : DotProduct  OutDataTypeStr=Inherit: Inherit via internal rule
  Sqrt : Sqrt  AlgorithmType=Newton-Raphson  SaturateOnIntegerOverflow=on
  l : Outport
  wires:
  Dot Product1/1 -> Sqrt/1
  L/1 -> Dot Product1/2, Dot Product1/1
  Sqrt/1 -> l/1  "Length"

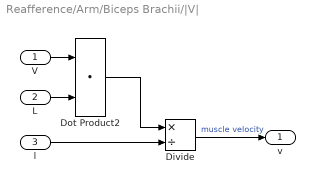
== system Reafference/Arm/Biceps Brachii/|V| ==
  V : Inport
  L : Inport  Port=2
  l : Inport  Port=3
  Divide : Product  Inputs=*/
  Dot Product2 : DotProduct  OutDataTypeStr=Inherit: Inherit via internal rule
  v : Outport
  wires:
  Dot Product2/1 -> Divide/1
  L/1 -> Dot Product2/2
  l/1 -> Divide/2
  V/1 -> Dot Product2/1
  Divide/1 -> v/1  "muscle velocity"

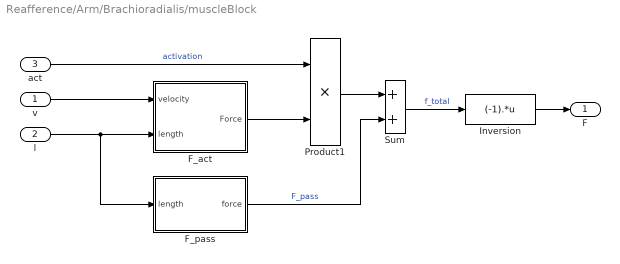
== system Reafference/Arm/Brachioradialis/muscleBlock ==
  v : Inport
  l : Inport  Port=2
  act : Inport  Port=3
  F_act : Subsystem  Description=active part of the force
  F_pass : Subsystem
  Inversion : MATLABFcn  MATLABFcn=(-1).*u
  Product1 : Product  RndMeth=Zero
  Sum : Sum
  F : Outport
  wires:
  v/1 -> F_act/1(velocity)
  l/1 -> F_pass/1(length), F_act/2(length)
  F_pass/1(force) -> Sum/2  "F_pass"
  Inversion/1 -> F/1
  Sum/1 -> Inversion/1  "f_total"
  Product1/1 -> Sum/1
  F_act/1(Force) -> Product1/2
  act/1 -> Product1/1  "activation"

== system Reafference/Arm/Brachioradialis/|L| ==
  L : Inport
  Dot Product1 : DotProduct  OutDataTypeStr=Inherit: Inherit via internal rule
  Sqrt : Sqrt  AlgorithmType=Newton-Raphson  SaturateOnIntegerOverflow=on
  l : Outport
  wires:
  Dot Product1/1 -> Sqrt/1
  L/1 -> Dot Product1/2, Dot Product1/1
  Sqrt/1 -> l/1  "Length"

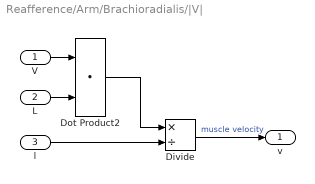
== system Reafference/Arm/Brachioradialis/|V| ==
  V : Inport
  L : Inport  Port=2
  l : Inport  Port=3
  Divide : Product  Inputs=*/
  Dot Product2 : DotProduct  OutDataTypeStr=Inherit: Inherit via internal rule
  v : Outport
  wires:
  Dot Product2/1 -> Divide/1
  L/1 -> Dot Product2/2
  l/1 -> Divide/2
  V/1 -> Dot Product2/1
  Divide/1 -> v/1  "muscle velocity"

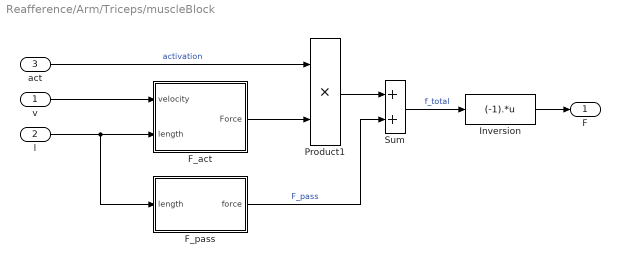
== system Reafference/Arm/Triceps/muscleBlock ==
  v : Inport
  l : Inport  Port=2
  act : Inport  Port=3
  F_act : Subsystem  Description=active part of the force
  F_pass : Subsystem
  Inversion : MATLABFcn  MATLABFcn=(-1).*u
  Product1 : Product  RndMeth=Zero
  Sum : Sum
  F : Outport
  wires:
  v/1 -> F_act/1(velocity)
  l/1 -> F_pass/1(length), F_act/2(length)
  F_pass/1(force) -> Sum/2  "F_pass"
  Inversion/1 -> F/1
  Sum/1 -> Inversion/1  "f_total"
  Product1/1 -> Sum/1
  F_act/1(Force) -> Product1/2
  act/1 -> Product1/1  "activation"

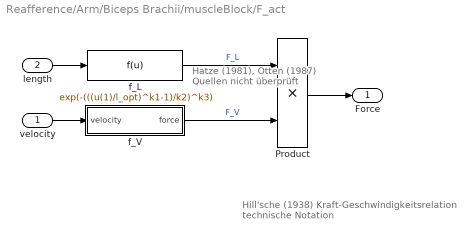
== system Reafference/Arm/Biceps Brachii/muscleBlock/F_act ==
  note: Hill'sche (1938) Kraft-Geschwindigkeitsrelation
      | technische Notation
  note: Hatze (1981), Otten (1987)
      | Quellen nicht überprüft
  velocity : Inport
  length : Inport  Port=2
  Product : Product  RndMeth=Zero
  f_L : Fcn  Expr=exp(-(((u(1)/l_opt)^k1-1)/k2)^k3)
  f_V : Subsystem
  Force : Outport
  wires:
  f_L/1 -> Product/1  "F_L"
  Product/1 -> Force/1
  f_V/1(force) -> Product/2  "F_V"
  length/1 -> f_L/1
  velocity/1 -> f_V/1(velocity)

== system Reafference/Arm/Biceps Brachii/muscleBlock/F_pass ==
  length : Inport
  f_pass_constrain : Fcn  Expr=f_max * exp((u-l_max)/lambda_max)
  force : Outport
  wires:
  length/1 -> f_pass_constrain/1
  f_pass_constrain/1 -> force/1  "f_pass_constrain"

== system Reafference/Arm/Brachioradialis/muscleBlock/F_act ==
  note: Hill'sche (1938) Kraft-Geschwindigkeitsrelation
      | technische Notation
  note: Hatze (1981), Otten (1987)
      | Quellen nicht überprüft
  velocity : Inport
  length : Inport  Port=2
  Product : Product  RndMeth=Zero
  f_L : Fcn  Expr=exp(-(((u(1)/l_opt)^k1-1)/k2)^k3)
  f_V : Subsystem
  Force : Outport
  wires:
  f_L/1 -> Product/1  "F_L"
  Product/1 -> Force/1
  f_V/1(force) -> Product/2  "F_V"
  length/1 -> f_L/1
  velocity/1 -> f_V/1(velocity)

== system Reafference/Arm/Brachioradialis/muscleBlock/F_pass ==
  length : Inport
  f_pass_constrain : Fcn  Expr=f_max * exp((u-l_max)/lambda_max)
  force : Outport
  wires:
  length/1 -> f_pass_constrain/1
  f_pass_constrain/1 -> force/1  "f_pass_constrain"

== system Reafference/Arm/Triceps/muscleBlock/F_act ==
  note: Hill'sche (1938) Kraft-Geschwindigkeitsrelation
      | technische Notation
  note: Hatze (1981), Otten (1987)
      | Quellen nicht überprüft
  velocity : Inport
  length : Inport  Port=2
  Product : Product  RndMeth=Zero
  f_L : Fcn  Expr=exp(-(((u(1)/l_opt)^k1-1)/k2)^k3)
  f_V : Subsystem
  Force : Outport
  wires:
  f_L/1 -> Product/1  "F_L"
  Product/1 -> Force/1
  f_V/1(force) -> Product/2  "F_V"
  length/1 -> f_L/1
  velocity/1 -> f_V/1(velocity)

== system Reafference/Arm/Triceps/muscleBlock/F_pass ==
  length : Inport
  f_pass_constrain : Fcn  Expr=f_max * exp((u-l_max)/lambda_max)
  force : Outport
  wires:
  length/1 -> f_pass_constrain/1
  f_pass_constrain/1 -> force/1  "f_pass_constrain"

== system Reafference/Arm/Biceps Brachii/muscleBlock/F_act/f_V ==
  velocity : Inport
  Compare To Zero : simulink/Logic and Bit Operations/Compare To Zero  relop=>=  OutDataTypeStr=uint8
  Index Vector : MultiPortSwitch  DataPortOrder=Zero-based contiguous  Inputs=2  zeroidx=on
  f_c : Fcn  Expr=c/(-u+b)-a
  f_e : Fcn  Expr=c_ecc/(-u-b_ecc)+a_ecc
  force : Outport
  wires:
  f_c/1 -> Index Vector/2
  f_e/1 -> Index Vector/3
  Compare To Zero/1 -> Index Vector/1
  velocity/1 -> f_e/1, f_c/1, Compare To Zero/1
  Index Vector/1 -> force/1

== system Reafference/Arm/Brachioradialis/muscleBlock/F_act/f_V ==
  velocity : Inport
  Compare To Zero : simulink/Logic and Bit Operations/Compare To Zero  relop=>=  OutDataTypeStr=uint8
  Index Vector : MultiPortSwitch  DataPortOrder=Zero-based contiguous  Inputs=2  zeroidx=on
  f_c : Fcn  Expr=c/(-u+b)-a
  f_e : Fcn  Expr=c_ecc/(-u-b_ecc)+a_ecc
  force : Outport
  wires:
  f_c/1 -> Index Vector/2
  f_e/1 -> Index Vector/3
  Compare To Zero/1 -> Index Vector/1
  velocity/1 -> f_e/1, f_c/1, Compare To Zero/1
  Index Vector/1 -> force/1

== system Reafference/Arm/Triceps/muscleBlock/F_act/f_V ==
  velocity : Inport
  Compare To Zero : simulink/Logic and Bit Operations/Compare To Zero  relop=>=  OutDataTypeStr=uint8
  Index Vector : MultiPortSwitch  DataPortOrder=Zero-based contiguous  Inputs=2  zeroidx=on
  f_c : Fcn  Expr=c/(-u+b)-a
  f_e : Fcn  Expr=c_ecc/(-u-b_ecc)+a_ecc
  force : Outport
  wires:
  f_c/1 -> Index Vector/2
  f_e/1 -> Index Vector/3
  Compare To Zero/1 -> Index Vector/1
  velocity/1 -> f_e/1, f_c/1, Compare To Zero/1
  Index Vector/1 -> force/1

== matlab function Reafference/Reservoir Learning/W_dot ==
  data: W_old input; W_new input; W_dot output; dt parameter
function W_dot = fcn(W_old, W_new, dt)
%#codegen

W = W_new-W_old;
W_dot = norm(W)/dt;

== matlab function Reafference/Arm/Drehmomentsumme ==
  data: lo input; y output; joint input
function y = fcn(lo,joint)
%#codegen
%-1000*(u(1)>=170)+1000*(u(1)<10)-0.01*u(2)
angle = joint(1)*180/pi;
omega = joint(2)*180/pi;
angle_min = 5;
angle_max = 165;
k = 200;
d = 0.04;

y = lo -k*(angle-angle_max)*(angle>=angle_max)-k*(angle-angle_min)*(angle<angle_min)-d*omega;

== matlab function Reafference/Reservoir Learning/Learning ==
  data: W input; q input; y input; h input; learn input; P input; W_out output; e output; P_out output
function [W_out, e, P_out] = fcn(W, q, y, h, learn, P)
%#eml

r = tanh(q);

e = y - h;
k = P*r;
c = 1/(1+r'*k);

W_out = W - learn*e*(k*c)';
P_out = P - k*(k'*c);

== matlab function Reafference/Reservoir Learning/Reservoir ==
  data: x input; tau parameter; I parameter; W input; q input; M parameter; F parameter; y output; qdot output
function [y,qdot] = fcn(x, tau, I, W, q, M, F)
%#eml

r = tanh(q);

y    = W*r;
qdot = 1/tau*(-q + I*x + M*r + F*y);
